simulink model "Design3"  (R2015a)
settings: Solver=ode45  StartTime=0.0  StopTime=1545  RelTol=1e-3
values from neighbouring files (symbols this model uses):
  C1 = 1E-7    (= 1e-07)    [Initialize.m]
  R0 = 1E9    (= 1000000000)    [Initialize.m]
  R1 = 1E8    (= 100000000)    [Initialize.m]
  R2 = 5E9    (= 5000000000)    [Initialize.m]
  R3 = 1E8    (= 100000000)    [Initialize.m]
libraries: fl_lib x10, nesl_utility x3, checkpacklib x1, simulink x1
settings Model: Creator=administrator  LastModifiedBy=administrator

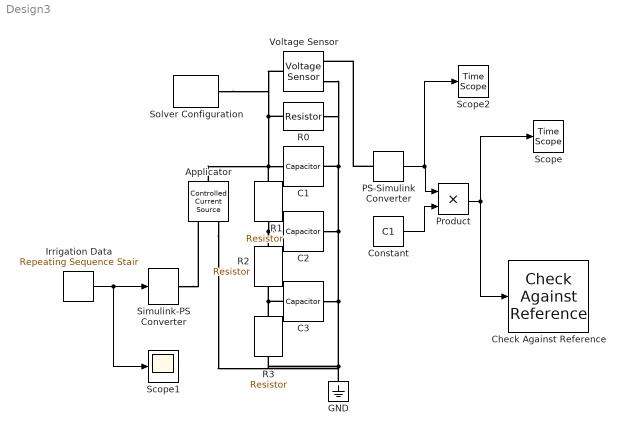
== system Design3 ==
  Applicator : fl_lib/Electrical/Electrical Sources/Controlled Current Source
  C1 : fl_lib/Electrical/Electrical Elements/Capacitor  c=C1 F  r=0 Ohm  g=0 1/Ohm  i_specify=off  i_priority=High  i=0 A  v_specify=off  v_priority=High  v=0 V  vc_specify=on  vc_priority=High  vc=V1 V
  C2 : fl_lib/Electrical/Electrical Elements/Capacitor  c=C2 F  r=0 Ohm  g=0 1/Ohm  i_specify=off  i_priority=High  i=0 A  v_specify=off  v_priority=High  v=0 V  vc_specify=on  vc_priority=High  vc=V2 V
  C3 : fl_lib/Electrical/Electrical Elements/Capacitor  c=C3 F  r=0 Ohm  g=0 1/Ohm  i_specify=off  i_priority=High  i=0 A  v_specify=off  v_priority=High  v=0 V  vc_specify=on  vc_priority=High  vc=V3 V
  Check Against Reference : checkpacklib/Check Against Reference  InstantiateOnLoad=on  enabled=on  stopWhenAssertionFail=off  export=off  ViewDlgPos=[100 200 510 390]  OpenViewOnLoad=off  LaunchViewOnOpen=on  TimeUnits=seconds  EnableReferenceBound=on  AbsTolerance=eps^(1/3)  RelTolerance=0.01  ReferenceTimes=[1:1060]  ReferenceAmplitudes=vwcT
  Constant : Constant  Value=C1
  GND : fl_lib/Electrical/Electrical Elements/Electrical Reference
  Irrigation Data : simulink/Sources/Repeating Sequence Stair  OutValues=IrrigationC  tsamp=1  OutMin=[]  OutMax=[]  OutDataTypeStr=double  OutputDataTypeScalingMode=double  OutDataType=fixdt(0,8)  ConRadixGroup=Best Precision: Vector-wise  OutScaling=2^-12
  PS-Simulink Converter : nesl_utility/PS-Simulink Converter  PhysicalDomain=network_engine_domain  SubClassName=ps_output  LeftPortType=input  RightPortType=output  PseudoPeriodic=off  Frequencies=[]  Unit=1  AffineConversion=off
  Product : Product
  R0 : fl_lib/Electrical/Electrical Elements/Resistor  R=R0 Ohm  i_specify=off  i_priority=High  i=0 A  v_specify=off  v_priority=High  v=0 V
  R1 : fl_lib/Electrical/Electrical Elements/Resistor  R=R1 Ohm  i_specify=off  i_priority=High  i=0 A  v_specify=off  v_priority=High  v=0 V
  R2 : fl_lib/Electrical/Electrical Elements/Resistor  R=R2 Ohm  i_specify=off  i_priority=High  i=0 A  v_specify=off  v_priority=High  v=0 V
  R3 : fl_lib/Electrical/Electrical Elements/Resistor  R=R3 Ohm  i_specify=off  i_priority=High  i=0 A  v_specify=off  v_priority=High  v=0 V
  Scope : TimeScope
  Scope1 : Scope
  Scope2 : TimeScope
  Simulink-PS Converter : nesl_utility/Simulink-PS Converter  PhysicalDomain=network_engine_domain  SubClassName=ps_input  LeftPortType=input  RightPortType=output  PseudoPeriodic=off  Frequencies=[]  NoiseDistribution=none  NoiseParameters=[]  Unit=1  AffineConversion=off  InputFiltering=off  SimscapeFilterOrder=1  InputFilterTimeConstant=0.001  UdotUserProvided=1
  Solver Configuration : nesl_utility/Solver Configuration  PhysicalDomain=network_engine_domain  SubClassName=solver  LeftPortType=input  RightPortType=generic  Accelerate=off  Tones=[]  Harmonics=[]  SimulateNoise=off  Profile=off  UseLocalSampling=off  EnableSwitchedLinearOptims=on  FrequencyDomain=off  UseCCode=off  RelTol=0.001  AbsTol=1e-06  MinStep=1e-09  ToWorkspace=off  RevertToSquareIcSolve=off  NumHomotopyIterations=100  DoDC=off  ResidualTolerance=1e-09  UseLocalSolver=off  LocalSolverChoice=NE_BACKWARD_EULER_ADVANCER  LocalSolverSampleTime=0.001  DoFixedCost=off  MaxNonlinIter=3  MaxModeIter=2  LinearAlgebra=Sparse  DelaysMemoryBudget=1024  AutomaticFiltering=on  FilteringTimeConstant=0.001
  Voltage Sensor : fl_lib/Electrical/Electrical Sensors/Voltage Sensor
  wires:
  Irrigation Data/1 -> Scope1/1, Simulink-PS Converter/1
  Constant/1 -> Product/2
  PS-Simulink Converter/1 -> Scope2/1, Product/1
  Product/1 -> Scope/1, Check Against Reference/1
  connections:
  C2/LConn1 -- R1/RConn1 -- R2/LConn1
  R1/LConn1 -- Solver Configuration/RConn1 -- Voltage Sensor/LConn1 -- R0/LConn1 -- C1/LConn1 -- Applicator/LConn1
  GND/LConn1 -- C2/RConn1 -- R0/RConn1 -- Voltage Sensor/RConn2 -- C1/RConn1 -- C3/RConn1 -- Applicator/RConn2 -- R3/RConn1
  R3/LConn1 -- C3/LConn1 -- R2/RConn1
  Simulink-PS Converter/RConn1 -- Applicator/RConn1
  PS-Simulink Converter/LConn1 -- Voltage Sensor/RConn1
